simulink library "lib5"  (R2020a)
settings: Solver=VariableStepAuto  StartTime=0.0  StopTime=10.0  RelTol=1e-3
undefined symbols (not defined in the file): L_lim
settings Model: Creator=hussein  LastModifiedBy=hussein

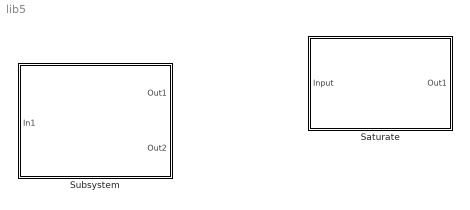
== system lib5 ==
  Saturate : Subsystem  mask{U_lim=0, L_lim=0, Value=L_lim}
      mask prompts: Value "Simulink:blkprm_prompts:ConstConstValue"
      mask Help: Hello
      mask TypeOptions Value: L_lim/Value | U_lim/Value
      mask DialogControl Value Prompt: Constant value:
      mask Display:
      | disp('Saturate');
      | color('red');
      | port_label('input',1,'signal');
      | port_label('output',1,'out');
  Subsystem : Subsystem  mask{GAIN=5}
      mask init:
      | if (GAIN>5)
      |     Thres = 0.1;
      | else
      |         Thres = 0.01;
      | end
      mask Help: abc
      mask Display:
      | disp('My_Block');
      | color('red');
      | port_label('input',1,'signal');
      | port_label('output',1,'out');
      | port_label('output',2,'Thres');

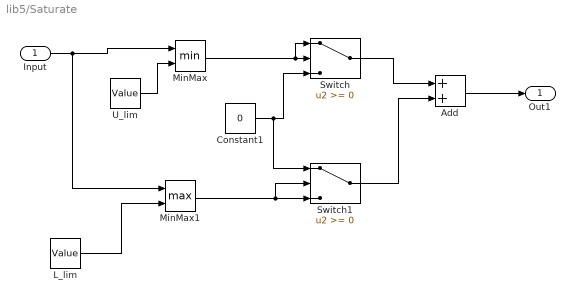
== system lib5/Saturate ==
  Input : Inport
  Add : Sum
  Constant1 : Constant  Value=0
  L_lim : Constant  Value=Value
  MinMax : MinMax  Inputs=2
  MinMax1 : MinMax  Function=max  Inputs=2
  Switch : Switch
  Switch1 : Switch
  U_lim : Constant  Value=Value
  Out1 : Outport
  wires:
  Input/1 -> MinMax1/1, MinMax/1
  U_lim/1 -> MinMax/2
  MinMax/1 -> Switch/1, Switch/2
  Constant1/1 -> Switch1/1, Switch/3
  Switch/1 -> Add/1
  L_lim/1 -> MinMax1/2
  MinMax1/1 -> Switch1/2, Switch1/3
  Switch1/1 -> Add/2
  Add/1 -> Out1/1

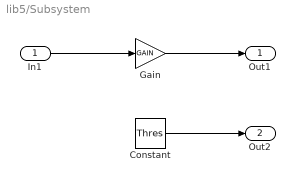
== system lib5/Subsystem ==
  In1 : Inport
  Constant : Constant  Value=Thres
  Gain : Gain  Gain=GAIN
  Out1 : Outport
  Out2 : Outport  Port=2
  wires:
  In1/1 -> Gain/1
  Gain/1 -> Out1/1
  Constant/1 -> Out2/1
